simulink model "pixhawk_sil_connector_example"  (R2023a)
settings: Solver=ode4  StartTime=0.0  StopTime=inf  FixedStep=0.004  RelTol=1e-3
model workspace (MAT data in the model file):
  sample_time = 0.004
undefined symbols (not defined in the file or in its folder): Earth, WGS84
libraries: simulink_extras x3, shared6dof x1, aerolibtransform2 x1, simulink x1, aerolibatmos2 x1, aerolibanimutils x1, sharedtransform x1, uavutilslib x1
settings Model: Creator=kboychev  LastModifiedBy=dferr
settings OptimizationCC: ZeroExternalMemoryAtStartup=off  ZeroInternalMemoryAtStartup=off
settings ModelReferenceCC: EnableRefExpFcnMdlSchedulingChecks=on
settings RTWCC: Toolchain=Microsoft Visual C++ 2017 v15.0 | nmake (64-bit Windows)  TargetLang=C++
settings GRTTargetCC: TargetLangStandard=C++11 (ISO)  CodeInterfacePackaging=C++ class

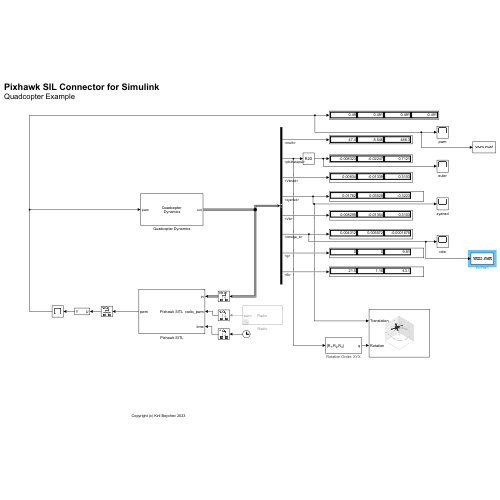
[thumbnail: Simulink's stored preview of the top-level diagram]
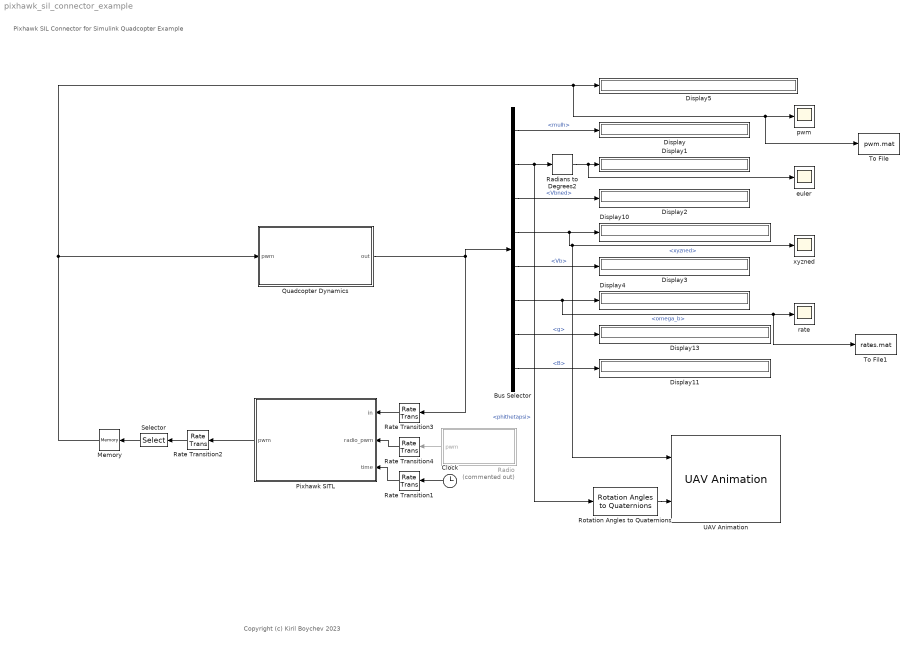
== system pixhawk_sil_connector_example ==
  note: Pixhawk SIL Connector for Simulink
      | Quadcopter Example
  note: Copyright (c) Kiril Boychev 2023
  Bus Selector : BusSelector  OutputSignals=mulh,phithetapsi,Vbned,xyzned,Vb,omega_b,g,B
  Clock : Clock
  Display{,1..5,10..11,13} (9 alike) : Display
  Memory : Memory  InitialCondition=[0 0 0 0]
  Pixhawk SITL : Subsystem
      mask Display:
      | fprintf('Pixhawk SITL');
      | port_label('input',1,'in');
      | port_label('input',2,'radio_pwm');
      | port_label('input',3,'time');
      | port_label('output',1,'pwm');
  Quadcopter Dynamics : Subsystem
      mask Display: fprintf('Quadcopter\n Dynamics');
  Radians to Degrees2 : simulink_extras/Transformations/Radians to Degrees
  Radio : Subsystem  Commented=on
      mask Display:
      | fprintf('Radio');
      | port_label('output',1,'pwm');
  Rate Transition{1..4} (4 alike) : RateTransition  OutPortSampleTime=sample_time
  Rotation Angles to Quaternions : sharedtransform/Rotation Angles to Quaternions  rotationOrder=XYX  aMode=aMode
  Selector : Selector  IndexMode=Zero-based  InputPortWidth=16  IndexOptions=Index vector (dialog)  Indices=[0:3]  OutputSizes=1
  To File : ToFile  Filename=pwm.mat  SaveFormat=Timeseries
  To File1 : ToFile  Filename=rates.mat  SaveFormat=Timeseries
  UAV Animation : uavutilslib/UAV Animation  UAVType=Multirotor  UAVSize=1  InertialZDirection=Down  SampleTime=-1
  euler : Scope
  pwm : Scope
  rate : Scope
  xyzned : Scope
  wires:
  Clock/1 -> Rate Transition1/1
  Radio/1(pwm) -> Rate Transition4/1
  Quadcopter Dynamics/1(out) -> Bus Selector/1, Rate Transition3/1
  Bus Selector/3 -> Display2/1  "<Vbned>"
  Bus Selector/1 -> Display/1  "<mulh>"
  Bus Selector/5 -> Display3/1  "<Vb>"
  Bus Selector/2 -> Rotation Angles to Quaternions/1, Radians to Degrees2/1  "<phithetapsi>"
  Bus Selector/8 -> Display11/1  "<B>"
  Radians to Degrees2/1 -> euler/1, Display1/1
  Bus Selector/7 -> Display13/1  "<g>"
  Bus Selector/4 -> UAV Animation/1, xyzned/1, Display10/1  "<xyzned>"
  Bus Selector/6 -> To File1/1, rate/1, Display4/1  "<omega_b>"
  Selector/1 -> Memory/1
  Pixhawk SITL/1(pwm) -> Rate Transition2/1
  Memory/1 -> To File/1, pwm/1, Display5/1, Quadcopter Dynamics/1(pwm)
  Rate Transition3/1 -> Pixhawk SITL/1(in)
  Rate Transition1/1 -> Pixhawk SITL/3(time)
  Rate Transition4/1 -> Pixhawk SITL/2(radio_pwm)
  Rate Transition2/1 -> Selector/1
  Rotation Angles to Quaternions/1 -> UAV Animation/2

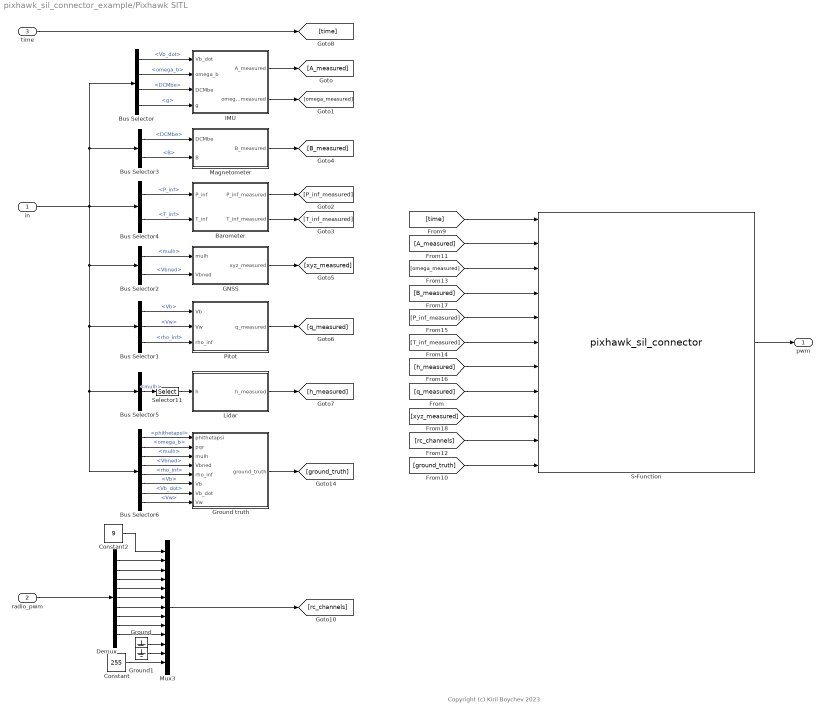
== system pixhawk_sil_connector_example/Pixhawk SITL ==
  note: Copyright (c) Kiril Boychev 2023
  in : Inport
  radio_pwm : Inport  Port=2
  time : Inport  Port=3
  Barometer : Subsystem
  Bus Selector : BusSelector  OutputSignals=Vb_dot,omega_b,DCMbe,g
  Bus Selector1 : BusSelector  OutputSignals=Vb,Vw,rho_inf
  Bus Selector2 : BusSelector  OutputSignals=mulh,Vbned
  Bus Selector3 : BusSelector  OutputSignals=DCMbe,B
  Bus Selector4 : BusSelector  OutputSignals=P_inf,T_inf
  Bus Selector5 : BusSelector  OutputSignals=mulh
  Bus Selector6 : BusSelector  OutputSignals=phithetapsi,omega_b,mulh,Vbned,rho_inf,Vb,Vb_dot,Vw
  Constant : Constant  Value=255
  Constant2 : Constant  Value=9
  Demux : Demux  Outputs=9
  GNSS : Subsystem
  Ground : Ground
  Ground truth : Subsystem
  Ground1 : Ground
  IMU : Subsystem
  Lidar : Subsystem
  Magnetometer : Subsystem
  Mux3 : Mux  Inputs=13
  Pitot : Subsystem
  S-Function : S-Function  FunctionName=pixhawk_sil_connector  SFunctionDeploymentMode=off  EnableBusSupport=off
  Selector11 : Selector  IndexMode=Zero-based  InputPortWidth=3  IndexOptions=Index vector (dialog)  Indices=2  OutputSizes=1
  pwm : Outport
  wires:
  IMU/1(A_measured) -> [A_measured]
  IMU/2(omega_b_measured) -> [omega_measured]
  Bus Selector4/1 -> Barometer/1(P_inf)  "<P_inf>"
  Bus Selector4/2 -> Barometer/2(T_inf)  "<T_inf>"
  Barometer/1(P_inf_measured) -> [P_inf_measured]
  Barometer/2(T_inf_measured) -> [T_inf_measured]
  Magnetometer/1(B_measured) -> [B_measured]
  Bus Selector2/1 -> GNSS/1(mulh)  "<mulh>"
  Constant/1 -> Mux3/13
  Constant2/1 -> Mux3/1
  Demux/9 -> Mux3/10
  Demux/8 -> Mux3/9
  Demux/7 -> Mux3/8
  Demux/6 -> Mux3/7
  Demux/5 -> Mux3/6
  Demux/4 -> Mux3/5
  Demux/3 -> Mux3/4
  Demux/2 -> Mux3/3
  Demux/1 -> Mux3/2
  Ground truth/1(ground_truth) -> [ground_truth]
  Bus Selector3/1 -> Magnetometer/1(DCMbe)  "<DCMbe>"
  Bus Selector3/2 -> Magnetometer/2(B)  "<B>"
  Bus Selector/1 -> IMU/1(Vb_dot)  "<Vb_dot>"
  Bus Selector/3 -> IMU/3(DCMbe)  "<DCMbe>"
  Bus Selector/4 -> IMU/4(g)  "<g>"
  Bus Selector/2 -> IMU/2(omega_b)  "<omega_b>"
  GNSS/1(xyz_measured) -> [xyz_measured]
  radio_pwm/1 -> Demux/1
  Bus Selector2/2 -> GNSS/2(Vbned)  "<Vbned>"
  [time] -> S-Function/1
  [rc_channels] -> S-Function/10
  [A_measured] -> S-Function/2
  [B_measured] -> S-Function/4
  [T_inf_measured] -> S-Function/6
  [q_measured] -> S-Function/8
  [xyz_measured] -> S-Function/9
  [omega_measured] -> S-Function/3
  [P_inf_measured] -> S-Function/5
  [h_measured] -> S-Function/7
  [ground_truth] -> S-Function/11
  time/1 -> [time]
  Mux3/1 -> [rc_channels]
  Bus Selector1/3 -> Pitot/3(rho_inf)  "<rho_inf>"
  Bus Selector1/1 -> Pitot/1(Vb)  "<Vb>"
  in/1 -> Bus Selector4/1, Bus Selector/1, Bus Selector3/1, Bus Selector1/1, Bus Selector5/1, Bus Selector6/1, Bus Selector2/1
  Bus Selector1/2 -> Pitot/2(Vw)  "<Vw>"
  Pitot/1(q_measured) -> [q_measured]
  S-Function/1 -> pwm/1
  Bus Selector6/1 -> Ground truth/1(phithetapsi)  "<phithetapsi>"
  Bus Selector6/2 -> Ground truth/2(pqr)  "<omega_b>"
  Bus Selector6/8 -> Ground truth/8(Vw)  "<Vw>"
  Bus Selector6/7 -> Ground truth/7(Vb_dot)  "<Vb_dot>"
  Bus Selector6/6 -> Ground truth/6(Vb)  "<Vb>"
  Bus Selector6/5 -> Ground truth/5(rho_inf)  "<rho_inf>"
  Bus Selector6/4 -> Ground truth/4(Vbned)  "<Vbned>"
  Bus Selector6/3 -> Ground truth/3(mulh)  "<mulh>"
  Lidar/1(h_measured) -> [h_measured]
  Bus Selector5/1 -> Selector11/1  "<mulh>"
  Selector11/1 -> Lidar/1(h)
  Ground/1 -> Mux3/11
  Ground1/1 -> Mux3/12

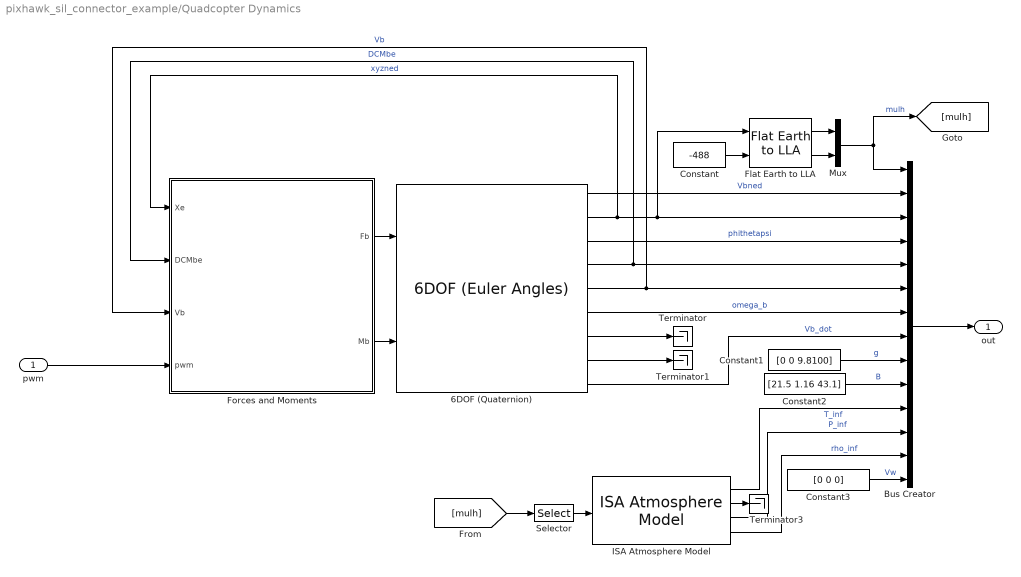
== system pixhawk_sil_connector_example/Quadcopter Dynamics ==
  pwm : Inport
  6DOF (Quaternion) : shared6dof/6DOF (Euler Angles)  units=Metric (MKS)  mtype=Fixed  rep=Quaternion  xme_0=[0 0 0]  Vm_0=[0 0 0]  eul_0=[0 0 0]  pm_0=[0 0 0]  mass_0=0.8  mass_e=0.5  mass_f=2.0  inertia=|  inertia_e=eye(3)  inertia_f=2*eye(3)  k_quat=1.0  vre_flag=on  abi_flag=on  aMode=0  xme_statename=''  Vm_statename=''  eul_statename=''  quat_statename=''  pm_statename=''  mass_statename=''
      | [    0.0050         0         0
      | ;         0    0.0050         0
      | ;         0         0    0.0090]
  Bus Creator : BusCreator  Inputs=14
  Constant : Constant  Value=-488
  Constant1 : Constant  Value=[0 0 9.8100]
  Constant2 : Constant  Value=[21.5 1.16 43.1]
  Constant3 : Constant  Value=[0 0 0]
  Flat Earth to LLA : aerolibtransform2/Flat Earth to LLA  units=Metric (MKS)  ptype=Earth (WGS84)  F=1/298.257223563  R=6378137  refPosPort=off  LL0=[47.3977 8.5456]  psi=0
  Forces and Moments : Subsystem
  ISA Atmosphere Model : aerolibatmos2/ISA Atmosphere Model  custom=off  g=9.80665  gamma=1.4  R=287.0531  L=0.0065  h_trop=11000  h_strat=20000  rho0=1.225  P0=101325  T0=288.15  h0=0
  Mux : Mux  Inputs=2
  Selector : Selector  IndexMode=Zero-based  InputPortWidth=3  IndexOptions=Index vector (dialog)  Indices=2  OutputSizes=1
  Terminator : Terminator
  Terminator1 : Terminator
  Terminator3 : Terminator
  out : Outport
  wires:
  pwm/1 -> Forces and Moments/4(pwm)
  Bus Creator/1 -> out/1
  Flat Earth to LLA/2 -> Mux/2
  Constant/1 -> Flat Earth to LLA/2
  Flat Earth to LLA/1 -> Mux/1
  6DOF (Quaternion)/2 -> Forces and Moments/1(Xe), Flat Earth to LLA/1, Bus Creator/3  "xyzned"
  6DOF (Quaternion)/4 -> Forces and Moments/2(DCMbe), Bus Creator/5  "DCMbe"
  6DOF (Quaternion)/5 -> Forces and Moments/3(Vb), Bus Creator/6  "Vb"
  Forces and Moments/1(Fb) -> 6DOF (Quaternion)/1
  Forces and Moments/2(Mb) -> 6DOF (Quaternion)/2
  6DOF (Quaternion)/1 -> Bus Creator/2  "Vbned"
  Mux/1 -> [mulh], Bus Creator/1  "mulh"
  6DOF (Quaternion)/3 -> Bus Creator/4  "phithetapsi"
  6DOF (Quaternion)/6 -> Bus Creator/7  "omega_b"
  6DOF (Quaternion)/7 -> Terminator/1
  6DOF (Quaternion)/8 -> Terminator1/1
  Constant1/1 -> Bus Creator/9  "g"
  Constant2/1 -> Bus Creator/10  "B"
  6DOF (Quaternion)/9 -> Bus Creator/8  "Vb_dot"
  ISA Atmosphere Model/1 -> Bus Creator/11  "T_inf"
  ISA Atmosphere Model/3 -> Bus Creator/12  "P_inf"
  [mulh] -> Selector/1
  Selector/1 -> ISA Atmosphere Model/1
  ISA Atmosphere Model/4 -> Bus Creator/13  "rho_inf"
  ISA Atmosphere Model/2 -> Terminator3/1
  Constant3/1 -> Bus Creator/14  "Vw"

== system pixhawk_sil_connector_example/Radio ==
  Mux : Mux  Inputs=9
  PWM Mapping : MATLAB Function  TreatAsAtomicUnit=on
  Pilot Joystick All : aerolibanimutils/Pilot Joystick  JoystickID=Joystick1  OutputConfiguration=AllOutputs  SampleTime=0.02
  Terminator : Terminator
  pwm : Outport
  wires:
  PWM Mapping/5(pwm5) -> Mux/5
  PWM Mapping/1(pwm1) -> Mux/1
  PWM Mapping/8(pwm8) -> Mux/8
  Mux/1 -> pwm/1
  PWM Mapping/7(pwm7) -> Mux/7
  PWM Mapping/9(pwm9) -> Mux/9
  PWM Mapping/3(pwm3) -> Mux/3
  PWM Mapping/4(pwm4) -> Mux/4
  PWM Mapping/6(pwm6) -> Mux/6
  PWM Mapping/2(pwm2) -> Mux/2
  Pilot Joystick All/3 -> Terminator/1
  Pilot Joystick All/2 -> PWM Mapping/2(buttons)
  Pilot Joystick All/1 -> PWM Mapping/1(analog)

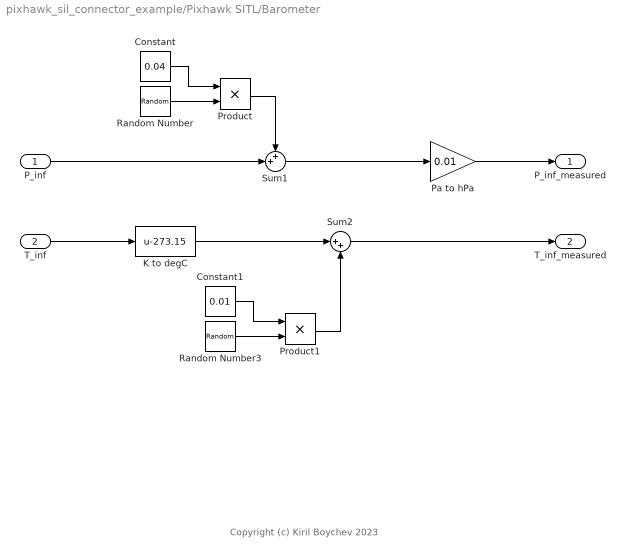
== system pixhawk_sil_connector_example/Pixhawk SITL/Barometer ==
  note: Copyright (c) Kiril Boychev 2023
  P_inf : Inport
  T_inf : Inport  Port=2
  Constant : Constant  Value=0.04
  Constant1 : Constant  Value=0.01
  K to degC : Bias  Bias=-273.15  SaturateOnIntegerOverflow=off
  Pa to hPa : Gain  Gain=0.01
  Product : Product
  Product1 : Product
  Random Number : RandomNumber  Seed=9  SampleTime=sample_time
  Random Number3 : RandomNumber  Seed=10  SampleTime=sample_time
  Sum1 : Sum  Inputs=++|
  Sum2 : Sum  Inputs=|++
  P_inf_measured : Outport
  T_inf_measured : Outport  Port=2
  wires:
  Sum1/1 -> Pa to hPa/1
  Random Number/1 -> Product/2
  Product/1 -> Sum1/1
  Constant/1 -> Product/1
  Sum2/1 -> T_inf_measured/1
  Random Number3/1 -> Product1/2
  Constant1/1 -> Product1/1
  Product1/1 -> Sum2/2
  T_inf/1 -> K to degC/1
  K to degC/1 -> Sum2/1
  P_inf/1 -> Sum1/2
  Pa to hPa/1 -> P_inf_measured/1

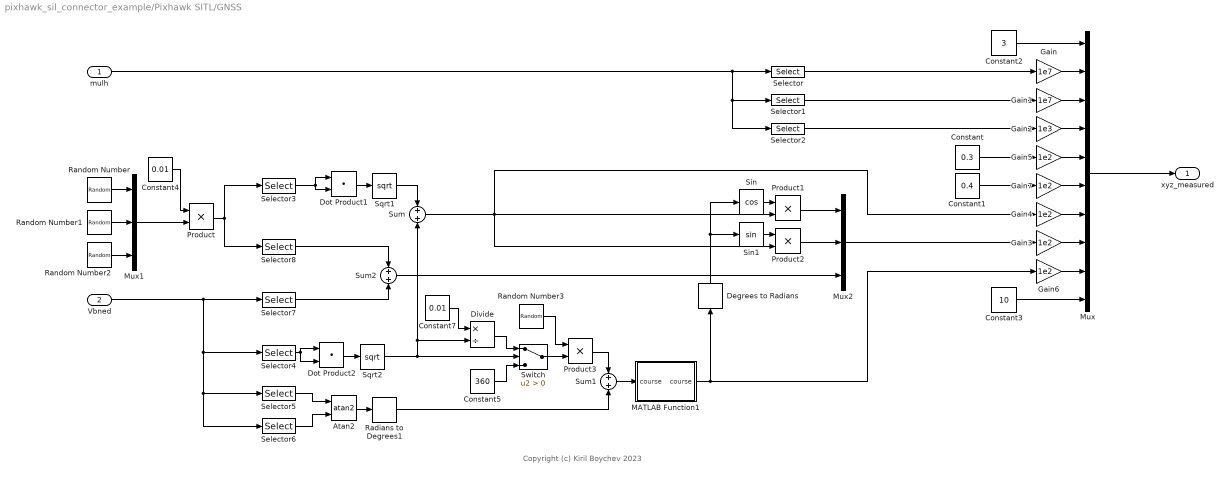
== system pixhawk_sil_connector_example/Pixhawk SITL/GNSS ==
  note: Copyright (c) Kiril Boychev 2023
  mulh : Inport
  Vbned : Inport  Port=2
  Atan2 : Trigonometry  Operator=atan2
  Constant : Constant  Value=0.3
  Constant1 : Constant  Value=0.4
  Constant2 : Constant  Value=3
  Constant3 : Constant  Value=10
  Constant4 : Constant  Value=0.01
  Constant5 : Constant  Value=360
  Constant7 : Constant  Value=0.01
  Degrees to Radians : simulink_extras/Transformations/Degrees to Radians
  Divide : Product  Inputs=*/
  Dot Product1 : DotProduct  OutDataTypeStr=Inherit: Inherit via internal rule
  Dot Product2 : DotProduct  OutDataTypeStr=Inherit: Inherit via internal rule
  Gain : Gain  Gain=1e7
  Gain1 : Gain  Gain=1e7
  Gain2 : Gain  Gain=1e3
  Gain{3..7} (5 alike) : Gain  Gain=1e2
  MATLAB Function1 : MATLAB Function  TreatAsAtomicUnit=on
  Mux : Mux  Inputs=10
  Mux1 : Mux  Inputs=3
  Mux2 : Mux  Inputs=3
  Product{,1..3} (4 alike) : Product
  Radians to Degrees1 : simulink_extras/Transformations/Radians to Degrees
  Random Number : RandomNumber  Seed=11  SampleTime=sample_time
  Random Number1 : RandomNumber  Seed=12  SampleTime=sample_time
  Random Number2 : RandomNumber  Seed=13  SampleTime=sample_time
  Random Number3 : RandomNumber  Seed=14  SampleTime=sample_time
  Selector : Selector  IndexMode=Zero-based  InputPortWidth=3  IndexOptions=Index vector (dialog)  Indices=0  OutputSizes=1
  Selector1 : Selector  IndexMode=Zero-based  InputPortWidth=3  IndexOptions=Index vector (dialog)  Indices=1  OutputSizes=1
  Selector2 : Selector  IndexMode=Zero-based  InputPortWidth=3  IndexOptions=Index vector (dialog)  Indices=2  OutputSizes=1
  Selector3 : Selector  IndexMode=Zero-based  InputPortWidth=3  IndexOptions=Index vector (dialog)  Indices=[0 1]  OutputSizes=1
  Selector4 : Selector  IndexMode=Zero-based  InputPortWidth=3  IndexOptions=Index vector (dialog)  Indices=[0 1]  OutputSizes=1
  Selector5 : Selector  IndexMode=Zero-based  InputPortWidth=3  IndexOptions=Index vector (dialog)  Indices=1  OutputSizes=1
  Selector6 : Selector  IndexMode=Zero-based  InputPortWidth=3  IndexOptions=Index vector (dialog)  Indices=0  OutputSizes=1
  Selector7 : Selector  IndexMode=Zero-based  InputPortWidth=3  IndexOptions=Index vector (dialog)  Indices=2  OutputSizes=1
  Selector8 : Selector  IndexMode=Zero-based  InputPortWidth=3  IndexOptions=Index vector (dialog)  Indices=2  OutputSizes=1
  Sin : Trigonometry  Operator=cos
  Sin1 : Trigonometry
  Sqrt1 : Sqrt
  Sqrt2 : Sqrt
  Sum : Sum
  Sum1 : Sum
  Sum2 : Sum
  Switch : Switch  Criteria=u2 > Threshold  SaturateOnIntegerOverflow=off  InputSameDT=off
  xyz_measured : Outport
  wires:
  mulh/1 -> Selector1/1, Selector2/1, Selector/1
  Selector/1 -> Gain/1
  Selector1/1 -> Gain1/1
  Selector2/1 -> Gain2/1
  Constant2/1 -> Mux/1
  Gain/1 -> Mux/2
  Gain1/1 -> Mux/3
  Gain2/1 -> Mux/4
  Constant/1 -> Gain5/1
  Constant1/1 -> Gain7/1
  Gain4/1 -> Mux/7
  Gain3/1 -> Mux/8
  Gain6/1 -> Mux/9
  Constant3/1 -> Mux/10
  Mux/1 -> xyz_measured/1
  Gain5/1 -> Mux/5
  Gain7/1 -> Mux/6
  Selector5/1 -> Atan2/1
  Sum2/1 -> Mux2/3
  Random Number1/1 -> Mux1/2
  Mux1/1 -> Product/2
  Atan2/1 -> Radians to Degrees1/1
  Constant4/1 -> Product/1
  Selector3/1 -> Dot Product1/1, Dot Product1/2
  Product/1 -> Selector3/1, Selector8/1
  Random Number/1 -> Mux1/1
  Switch/1 -> Product3/2
  Sum/1 -> Product2/2, Gain4/1, Product1/2
  Constant7/1 -> Divide/1
  Sqrt2/1 -> Switch/2, Divide/2, Sum/2
  Random Number2/1 -> Mux1/3
  Selector4/1 -> Dot Product2/1, Dot Product2/2
  Dot Product1/1 -> Sqrt1/1
  Sin/1 -> Product1/1
  Random Number3/1 -> Product3/1
  Degrees to Radians/1 -> Sin/1, Sin1/1
  Divide/1 -> Switch/1
  Selector6/1 -> Atan2/2
  Sin1/1 -> Product2/1
  Sum1/1 -> MATLAB Function1/1("course ")
  Dot Product2/1 -> Sqrt2/1
  Radians to Degrees1/1 -> Sum1/2
  Product3/1 -> Sum1/1
  MATLAB Function1/1(course) -> Degrees to Radians/1, Gain6/1
  Constant5/1 -> Switch/3
  Product1/1 -> Mux2/1
  Product2/1 -> Mux2/2
  Mux2/1 -> Gain3/1
  Sqrt1/1 -> Sum/1
  Selector7/1 -> Sum2/2
  Selector8/1 -> Sum2/1
  Vbned/1 -> Selector6/1, Selector5/1, Selector4/1, Selector7/1

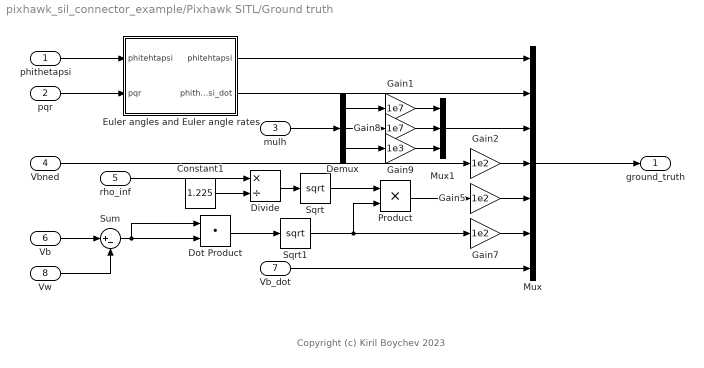
== system pixhawk_sil_connector_example/Pixhawk SITL/Ground truth ==
  note: Copyright (c) Kiril Boychev 2023
  phithetapsi : Inport
  pqr : Inport  Port=2
  mulh : Inport  Port=3
  Vbned : Inport  Port=4
  rho_inf : Inport  Port=5
  Vb : Inport  Port=6
  Vb_dot : Inport  Port=7
  Vw : Inport  Port=8
  Constant1 : Constant  Value=1.225
  Demux : Demux  Outputs=3
  Divide : Product  Inputs=*/
  Dot Product : DotProduct  OutDataTypeStr=Inherit: Inherit via internal rule
  Euler angles and Euler angle rates : MATLAB Function  TreatAsAtomicUnit=on
  Gain1 : Gain  Gain=1e7
  Gain2 : Gain  Gain=1e2
  Gain5 : Gain  Gain=1e2
  Gain7 : Gain  Gain=1e2
  Gain8 : Gain  Gain=1e7
  Gain9 : Gain  Gain=1e3
  Mux : Mux  Inputs=7
  Mux1 : Mux  Inputs=3
  Product : Product
  Sqrt : Sqrt
  Sqrt1 : Sqrt
  Sum : Sum  Inputs=|+-
  ground_truth : Outport
  wires:
  Vbned/1 -> Gain2/1
  Mux/1 -> ground_truth/1
  Gain5/1 -> Mux/5
  Gain7/1 -> Mux/6
  mulh/1 -> Demux/1
  Demux/1 -> Gain1/1
  Demux/2 -> Gain8/1
  Demux/3 -> Gain9/1
  Gain1/1 -> Mux1/1
  Gain8/1 -> Mux1/2
  Gain9/1 -> Mux1/3
  Mux1/1 -> Mux/3
  Gain2/1 -> Mux/4
  Product/1 -> Gain5/1
  Vb_dot/1 -> Mux/7
  Euler angles and Euler angle rates/2(phithetapsi_dot) -> Mux/2
  Euler angles and Euler angle rates/1(phitehtapsi) -> Mux/1
  pqr/1 -> Euler angles and Euler angle rates/2(pqr)
  phithetapsi/1 -> Euler angles and Euler angle rates/1("phitehtapsi ")
  Sqrt1/1 -> Gain7/1, Product/2
  Sum/1 -> Dot Product/1, Dot Product/2
  Divide/1 -> Sqrt/1
  Constant1/1 -> Divide/2
  rho_inf/1 -> Divide/1
  Sqrt/1 -> Product/1
  Dot Product/1 -> Sqrt1/1
  Vb/1 -> Sum/1
  Vw/1 -> Sum/2

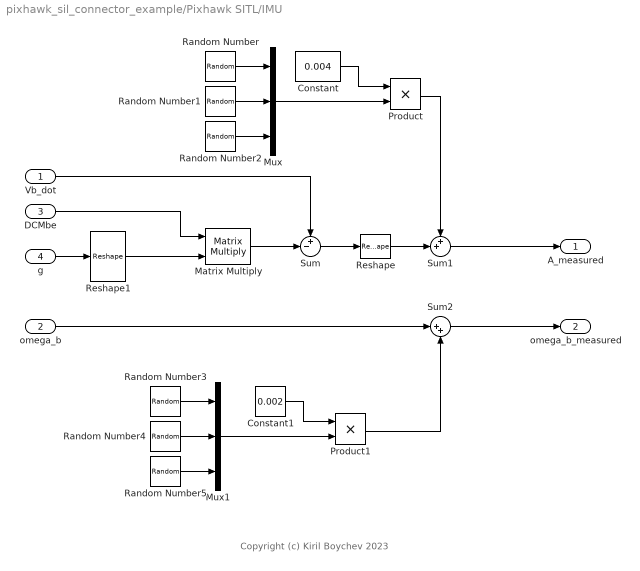
== system pixhawk_sil_connector_example/Pixhawk SITL/IMU ==
  note: Copyright (c) Kiril Boychev 2023
  Vb_dot : Inport
  omega_b : Inport  Port=2
  DCMbe : Inport  Port=3
  g : Inport  Port=4
  Constant : Constant  Value=0.004
  Constant1 : Constant  Value=0.002
  Matrix Multiply : Product  Multiplication=Matrix(*)
  Mux : Mux  Inputs=3
  Mux1 : Mux  Inputs=3
  Product : Product
  Product1 : Product
  Random Number : RandomNumber  SampleTime=sample_time
  Random Number1 : RandomNumber  Seed=1  SampleTime=sample_time
  Random Number2 : RandomNumber  Seed=2  SampleTime=sample_time
  Random Number3 : RandomNumber  Seed=3  SampleTime=sample_time
  Random Number4 : RandomNumber  Seed=4  SampleTime=sample_time
  Random Number5 : RandomNumber  Seed=5  SampleTime=sample_time
  Reshape : Reshape
  Reshape1 : Reshape  OutputDimensionality=Column vector (2-D)
  Sum : Sum  Inputs=+-|
  Sum1 : Sum  Inputs=++|
  Sum2 : Sum  Inputs=|++
  A_measured : Outport
  omega_b_measured : Outport  Port=2
  wires:
  g/1 -> Reshape1/1
  DCMbe/1 -> Matrix Multiply/1
  Matrix Multiply/1 -> Sum/2
  Vb_dot/1 -> Sum/1
  Reshape1/1 -> Matrix Multiply/2
  Sum/1 -> Reshape/1
  Sum1/1 -> A_measured/1
  Random Number1/1 -> Mux/2
  Random Number/1 -> Mux/1
  Random Number2/1 -> Mux/3
  Mux/1 -> Product/2
  Product/1 -> Sum1/1
  Constant/1 -> Product/1
  Sum2/1 -> omega_b_measured/1
  Mux1/1 -> Product1/2
  Random Number4/1 -> Mux1/2
  Random Number3/1 -> Mux1/1
  Random Number5/1 -> Mux1/3
  Constant1/1 -> Product1/1
  Product1/1 -> Sum2/2
  omega_b/1 -> Sum2/1
  Reshape/1 -> Sum1/2

== system pixhawk_sil_connector_example/Pixhawk SITL/Lidar ==
  note: Copyright (c) Kiril Boychev 2023
  h : Inport
  Bias : Bias  Bias=-488  SaturateOnIntegerOverflow=off
  Constant1 : Constant  Value=0.005
  Product2 : Product
  Random Number1 : RandomNumber  Seed=16  SampleTime=sample_time
  Sum3 : Sum  Inputs=|++
  m to cm : Gain  Gain=1e2
  h_measured : Outport
  wires:
  Constant1/1 -> Product2/1
  Product2/1 -> Sum3/2
  Random Number1/1 -> Product2/2
  h/1 -> Bias/1
  Bias/1 -> Sum3/1
  Sum3/1 -> m to cm/1
  m to cm/1 -> h_measured/1

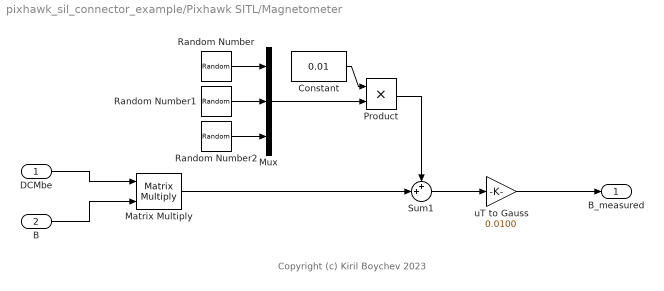
== system pixhawk_sil_connector_example/Pixhawk SITL/Magnetometer ==
  note: Copyright (c) Kiril Boychev 2023
  DCMbe : Inport
  B : Inport  Port=2
  Constant : Constant  Value=0.01
  Matrix Multiply : Product  Multiplication=Matrix(*)
  Mux : Mux  Inputs=3
  Product : Product
  Random Number : RandomNumber  Seed=6  SampleTime=sample_time
  Random Number1 : RandomNumber  Seed=7  SampleTime=sample_time
  Random Number2 : RandomNumber  Seed=8  SampleTime=sample_time
  Sum1 : Sum  Inputs=++|
  uT to Gauss : Gain  Gain=0.0100
  B_measured : Outport
  wires:
  Product/1 -> Sum1/1
  Random Number1/1 -> Mux/2
  Mux/1 -> Product/2
  Random Number/1 -> Mux/1
  Constant/1 -> Product/1
  Random Number2/1 -> Mux/3
  Matrix Multiply/1 -> Sum1/2
  DCMbe/1 -> Matrix Multiply/1
  Sum1/1 -> uT to Gauss/1
  B/1 -> Matrix Multiply/2
  uT to Gauss/1 -> B_measured/1

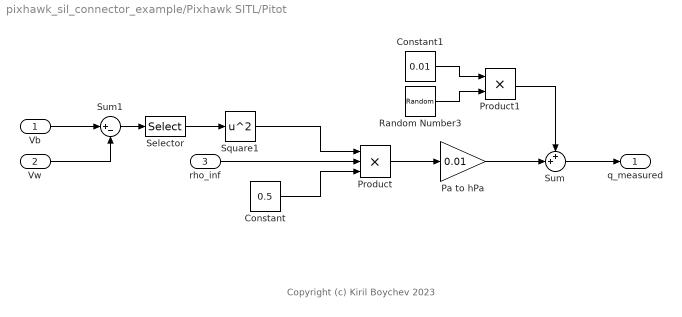
== system pixhawk_sil_connector_example/Pixhawk SITL/Pitot ==
  note: Copyright (c) Kiril Boychev 2023
  Vb : Inport
  Vw : Inport  Port=2
  rho_inf : Inport  Port=3
  Constant : Constant  Value=0.5
  Constant1 : Constant  Value=0.01
  Pa to hPa : Gain  Gain=0.01
  Product : Product  Inputs=3
  Product1 : Product
  Random Number3 : RandomNumber  Seed=15  SampleTime=sample_time
  Selector : Selector  IndexMode=Zero-based  InputPortWidth=3  IndexOptions=Index vector (dialog)  Indices=0  OutputSizes=1
  Square1 : Math  Operator=square
  Sum : Sum  Inputs=++|
  Sum1 : Sum  Inputs=|+-
  q_measured : Outport
  wires:
  Product1/1 -> Sum/1
  Random Number3/1 -> Product1/2
  Constant1/1 -> Product1/1
  Pa to hPa/1 -> Sum/2
  Sum/1 -> q_measured/1
  Selector/1 -> Square1/1
  Square1/1 -> Product/1
  rho_inf/1 -> Product/2
  Constant/1 -> Product/3
  Product/1 -> Pa to hPa/1
  Vw/1 -> Sum1/2
  Vb/1 -> Sum1/1
  Sum1/1 -> Selector/1

== system pixhawk_sil_connector_example/Quadcopter Dynamics/Forces and Moments ==
  Xe : Inport
  DCMbe : Inport  Port=2
  Vb : Inport  Port=3
  pwm : Inport  Port=4
  Add : Sum  Inputs=++++
  Drag Force : Subsystem
  Gravity : Subsystem
  Normal Force : Subsystem
  Rotor Forces and Moments : Subsystem
  Fb : Outport
  Mb : Outport  Port=2
  wires:
  pwm/1 -> Rotor Forces and Moments/1(pwm)
  DCMbe/1 -> Drag Force/1(DCMbe), Gravity/1(DCM_be)
  Gravity/1(Fb) -> Add/1
  Add/1 -> Fb/1
  Rotor Forces and Moments/2(Mb) -> Mb/1
  Vb/1 -> Drag Force/2(Vb), Normal Force/1(Vb)
  Rotor Forces and Moments/1(Fb) -> Add/2
  Drag Force/1(Fb) -> Add/3
  Normal Force/1(Fb) -> Add/4
  Xe/1 -> Normal Force/2(Xe)

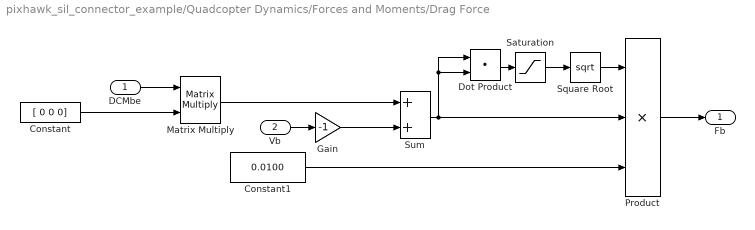
== system pixhawk_sil_connector_example/Quadcopter Dynamics/Forces and Moments/Drag Force ==
  DCMbe : Inport
  Vb : Inport  Port=2
  Constant : Constant  Value=[ 0 0 0]
  Constant1 : Constant  Value=0.0100
  Dot Product : DotProduct  OutDataTypeStr=Inherit: Inherit via internal rule
  Gain : Gain  Gain=-1
  Matrix Multiply : Product  Multiplication=Matrix(*)
  Product : Product  Inputs=3
  Saturation : Saturate  UpperLimit=inf  LowerLimit=0.0001
  Square Root : Sqrt
  Sum : Sum
  Fb : Outport
  wires:
  Sum/1 -> Dot Product/2, Dot Product/1, Product/2
  DCMbe/1 -> Matrix Multiply/1
  Product/1 -> Fb/1
  Saturation/1 -> Square Root/1
  Vb/1 -> Gain/1
  Dot Product/1 -> Saturation/1
  Square Root/1 -> Product/1
  Matrix Multiply/1 -> Sum/1
  Gain/1 -> Sum/2
  Constant1/1 -> Product/3
  Constant/1 -> Matrix Multiply/2

== system pixhawk_sil_connector_example/Quadcopter Dynamics/Forces and Moments/Gravity ==
  DCM_be : Inport
  Constant : Constant  Value=[0 0 9.8100]'
  Gain : Gain  Gain=0.8
  Matrix Multiply : Product  Multiplication=Matrix(*)
  Fb : Outport
  wires:
  Matrix Multiply/1 -> Gain/1
  Constant/1 -> Matrix Multiply/2
  DCM_be/1 -> Matrix Multiply/1
  Gain/1 -> Fb/1

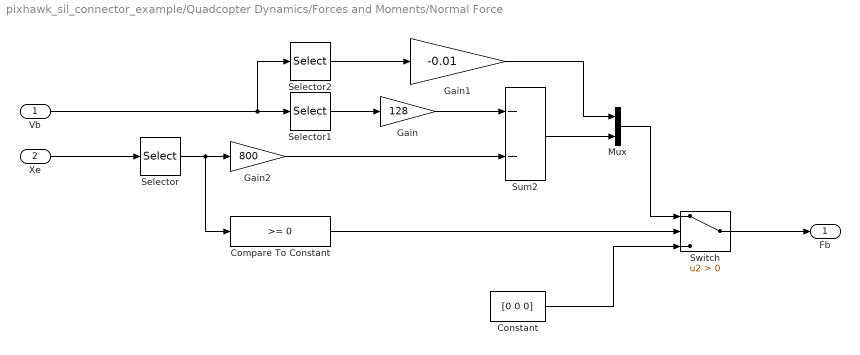
== system pixhawk_sil_connector_example/Quadcopter Dynamics/Forces and Moments/Normal Force ==
  Vb : Inport
  Xe : Inport  Port=2
  Compare To Constant : simulink/Logic and Bit Operations/Compare To Constant  relop=>=  const=0  OutDataTypeStr=boolean
  Constant : Constant  Value=[0 0 0]  SampleTime=-1
  Gain : Gain  Gain=128  SaturateOnIntegerOverflow=on  OutDataTypeStr=Inherit: Same as input  ParamDataTypeStr=Inherit: Same as input
  Gain1 : Gain  Gain=-0.01
  Gain2 : Gain  Gain=800  SaturateOnIntegerOverflow=on  OutDataTypeStr=Inherit: Same as input  ParamDataTypeStr=Inherit: Same as input
  Mux : Mux  Inputs=2
  Selector : Selector  InputPortWidth=3  IndexOptions=Index vector (dialog)  Indices=[3]  OutputSizes=1
  Selector1 : Selector  InputPortWidth=3  IndexOptions=Index vector (dialog)  Indices=[3]  OutputSizes=1
  Selector2 : Selector  InputPortWidth=3  IndexOptions=Index vector (dialog)  Indices=[1 2]  OutputSizes=1
  Sum2 : Sum  Inputs=--  InputSameDT=on  SaturateOnIntegerOverflow=on  OutDataTypeStr=Inherit: Same as first input
  Switch : Switch  Criteria=u2 > Threshold  SaturateOnIntegerOverflow=off  InputSameDT=off
  Fb : Outport
  wires:
  Selector/1 -> Gain2/1, Compare To Constant/1
  Gain2/1 -> Sum2/2
  Gain/1 -> Sum2/1
  Sum2/1 -> Mux/2
  Xe/1 -> Selector/1
  Compare To Constant/1 -> Switch/2
  Selector1/1 -> Gain/1
  Vb/1 -> Selector2/1, Selector1/1
  Constant/1 -> Switch/3
  Gain1/1 -> Mux/1
  Selector2/1 -> Gain1/1
  Mux/1 -> Switch/1
  Switch/1 -> Fb/1

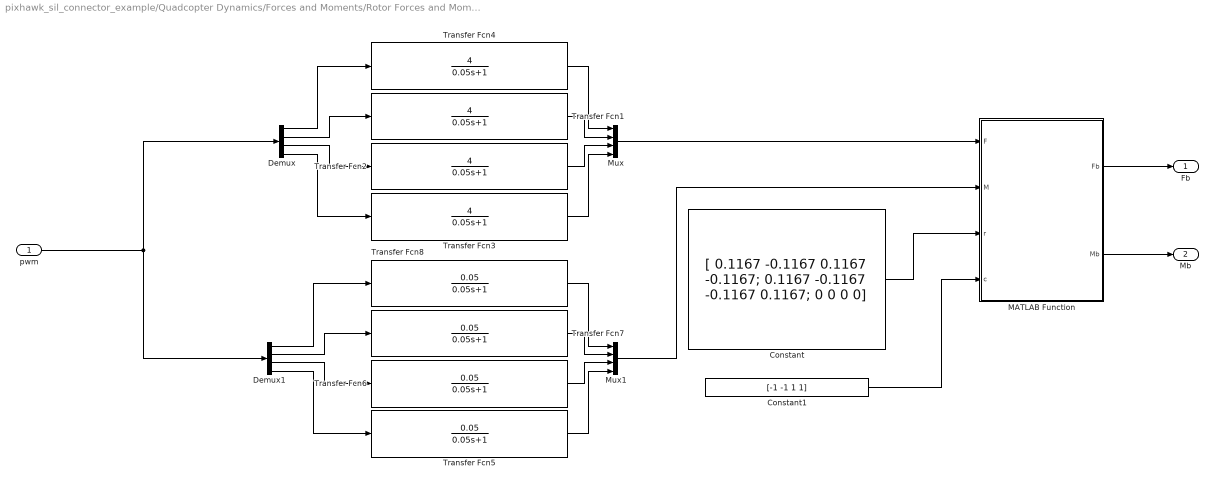
== system pixhawk_sil_connector_example/Quadcopter Dynamics/Forces and Moments/Rotor Forces and Moments ==
  pwm : Inport
  Constant : Constant  Value=|
      | [    0.1167   -0.1167    0.1167   -0.1167;
      |     0.1167   -0.1167   -0.1167    0.1167;
      |          0         0         0         0]
  Constant1 : Constant  Value=[-1 -1 1 1]
  Demux : Demux
  Demux1 : Demux
  MATLAB Function : MATLAB Function  TreatAsAtomicUnit=on
  Mux : Mux
  Mux1 : Mux
  Transfer Fcn{1..4} (4 alike) : TransferFcn  Numerator=[4]  Denominator=[0.05 1]
  Transfer Fcn{5..8} (4 alike) : TransferFcn  Numerator=[0.05]  Denominator=[0.05 1]
  Fb : Outport
  Mb : Outport  Port=2
  wires:
  MATLAB Function/1(Fb) -> Fb/1
  MATLAB Function/2(Mb) -> Mb/1
  Constant/1 -> MATLAB Function/3(r)
  Constant1/1 -> MATLAB Function/4(c)
  Mux1/1 -> MATLAB Function/2(M)
  Mux/1 -> MATLAB Function/1(F)
  Transfer Fcn4/1 -> Mux/1
  Demux/1 -> Transfer Fcn4/1
  Transfer Fcn3/1 -> Mux/4
  Transfer Fcn1/1 -> Mux/2
  Demux/3 -> Transfer Fcn2/1
  Demux/2 -> Transfer Fcn1/1
  Transfer Fcn2/1 -> Mux/3
  Demux/4 -> Transfer Fcn3/1
  Transfer Fcn8/1 -> Mux1/1
  Demux1/1 -> Transfer Fcn8/1
  pwm/1 -> Demux1/1, Demux/1
  Transfer Fcn5/1 -> Mux1/4
  Transfer Fcn7/1 -> Mux1/2
  Demux1/3 -> Transfer Fcn6/1
  Demux1/2 -> Transfer Fcn7/1
  Transfer Fcn6/1 -> Mux1/3
  Demux1/4 -> Transfer Fcn5/1

== matlab function pixhawk_sil_connector_example/Quadcopter Dynamics/Forces and Moments/Rotor Forces and Moments/MATLAB Function ==
  data: F input; M input; r input; Fb output; Mb output; c input
function [Fb, Mb] = forces_and_moments(F, M, r, c)
%#codegen
Fx = 0;
Fy = 0;
Fz = -sum(F);

Fb = [Fx; Fy; Fz];

Mb = [0; 0; 0];

for i = 1:4
    ri = r(:, i);
    Fi = [0, 0, -F(i)]';
    Mb = Mb +  cross(ri, Fi);
    Mb(3) = Mb(3) - c(i)*M(i); 
end

end

== matlab function pixhawk_sil_connector_example/Radio/PWM Mapping ==
  data: analog input; pwm1 output; pwm2 output; pwm3 output; pwm4 output; pwm5 output; buttons input; pwm6 output; pwm7 output; pwm8 output; pwm9 output
function [pwm1,pwm2,pwm3,pwm4,pwm5,pwm6,pwm7,pwm8,pwm9] = pmw_mapping(analog,buttons)

analog=round(analog*100)/100;
pwm1=(analog(1)+1)*500+1000;
pwm2=(analog(2)+1)*500+1000;
pwm3=analog(3)*1000+1000;
pwm4=(analog(4)+1)*500+1000;
pwm5=1000;
pwm6=1000;
pwm7=1000;
pwm8=1000;
pwm9=1000;

if buttons==1
    pwm5=2000;
elseif buttons==16
    pwm6=2000;
elseif buttons==32
    pwm7=2000;
elseif buttons==64
    pwm8=2000;
elseif buttons==128
    pwm9=2000;
end

== matlab function pixhawk_sil_connector_example/Pixhawk SITL/GNSS/MATLAB Function1 ==
  data: course input; course output
function course = wrapToMaxCourse(course)

    isPositive = (course > 0);
    course = mod(course, 360);
    course((course == 0) & isPositive) = 360;

end

== matlab function pixhawk_sil_connector_example/Pixhawk SITL/Ground truth/Euler angles and Euler angle rates ==
  data: phitehtapsi output; phitehtapsi input; phithetapsi_dot output; pqr input
function [phitehtapsi,phithetapsi_dot] = euler_angle_rates(phitehtapsi,pqr)
    
    phi=phitehtapsi(1);
    theta=phitehtapsi(2);

    sphi=sin(phi);
    cphi=cos(phi);
    stheta=sin(theta);
    ctheta=cos(theta);

    phithetapsi_dot=[1,sphi*stheta/ctheta,cphi*stheta/ctheta;
        0,cphi,-sphi;
        0,sphi/ctheta,cphi/ctheta]*pqr;
